simulink model "send_a429_r2019b"  (R2019b)
settings: Solver=VariableStepAuto  StartTime=0.0  StopTime=10.0  RelTol=1e-3
PreLoadFcn:
  | ds = Simulink.SimulationData.Dataset();
  | ds = ds.addElement(timeseries(uint8((1:11)' + (1:4)),       (0:10)', 'Name', 'AnA429SamplingMessage'),   'Name', 'AnA429SamplingMessage');
  | ds = ds.addElement(timeseries(uint8((250:-1:240)' + (1:4)), (0:10)', 'Name', 'AnA429QueuingMessage'),    'Name', 'AnA429QueuingMessage');
model workspace (MAT data in the model file):
  ED247Configuration(1).name = 'T11M4_A429_SIMU2SWIM_BUS_1_350_10_I'
  ED247Configuration(1).direction = 'OUT'
  ED247Configuration(1).type = 'uint8'
  ED247Configuration(1).dimensions = 1
  ED247Configuration(1).width = 4
  ED247Configuration(1).size = 4
  ED247Configuration(1).sample_time = 1
  ED247Configuration(1).validity_duration = 0
  ED247Configuration(1).signal_type = 'A429'
  ED247Configuration(1).sample_size = 4
  ED247Configuration(2).name = 'T11M4_A429_SIMU2SWIM_BUS_1_200_10_I'
  ED247Configuration(2).direction = 'OUT'
  ED247Configuration(2).type = 'uint8'
  ED247Configuration(2).dimensions = 1
  ED247Configuration(2).width = 4
  ED247Configuration(2).size = 4
  ED247Configuration(2).sample_time = 1
  ED247Configuration(2).validity_duration = 0
  ED247Configuration(2).signal_type = 'A429'
  ED247Configuration(2).sample_size = 4
  ED247Configuration(3).name = 'T11M4_A429_SIMU2SWIM_BUS_1_200_11_I'
  ED247Configuration(3).direction = 'OUT'
  ED247Configuration(3).type = 'uint8'
  ED247Configuration(3).dimensions = 1
  ED247Configuration(3).width = 4
  ED247Configuration(3).size = 4
  ED247Configuration(3).sample_time = 1
  ED247Configuration(3).validity_duration = 0
  ED247Configuration(3).signal_type = 'A429'
  ED247Configuration(3).sample_size = 4
libraries: lib_ed247 x2
settings Model: EnablePacing=on  Creator=odufour  LastModifiedBy=odufour
settings DataIOCC: ExternalInput=ds  LoadExternalInput=on

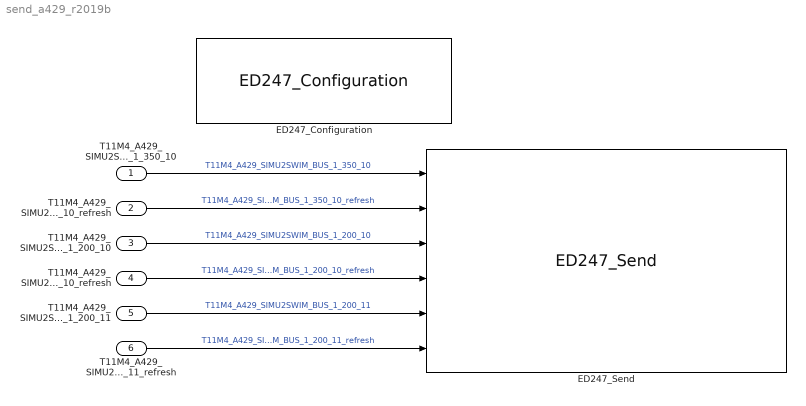
== system send_a429_r2019b ==
  T11M4_A429_SIMU2SWIM_BUS_1_350_10 : Inport  OutDataTypeStr=uint8  PortDimensions=4  SampleTime=0.1
  T11M4_A429_SIMU2SWIM_BUS_1_350_10_refresh : Inport  Port=2  OutDataTypeStr=boolean
  T11M4_A429_SIMU2SWIM_BUS_1_200_10 : Inport  Port=3  OutDataTypeStr=uint8  PortDimensions=4  SampleTime=0.1
  T11M4_A429_SIMU2SWIM_BUS_1_200_10_refresh : Inport  Port=4  OutDataTypeStr=boolean
  T11M4_A429_SIMU2SWIM_BUS_1_200_11 : Inport  Port=5  OutDataTypeStr=uint8  PortDimensions=4  SampleTime=0.1
  T11M4_A429_SIMU2SWIM_BUS_1_200_11_refresh : Inport  Port=6  OutDataTypeStr=boolean
  ED247_Configuration : lib_ed247/ED247_Configuration  configurationFilename='ecic_func_exchange_a429_uc_main_simple.xml'  enableLog=off  logFilename=''
      settings: SourceProductName=Airbus ED247
  ED247_Send : lib_ed247/ED247_Send  enable_refresh=on  show_port_labels=on
      settings: SourceProductName=Airbus ED247
  wires:
  T11M4_A429_SIMU2SWIM_BUS_1_350_10/1 -> ED247_Send/1  "T11M4_A429_SIMU2SWIM_BUS_1_350_10"
  T11M4_A429_SIMU2SWIM_BUS_1_350_10_refresh/1 -> ED247_Send/2  "T11M4_A429_SIMU2SWIM_BUS_1_350_10_refresh"
  T11M4_A429_SIMU2SWIM_BUS_1_200_10/1 -> ED247_Send/3  "T11M4_A429_SIMU2SWIM_BUS_1_200_10"
  T11M4_A429_SIMU2SWIM_BUS_1_200_10_refresh/1 -> ED247_Send/4  "T11M4_A429_SIMU2SWIM_BUS_1_200_10_refresh"
  T11M4_A429_SIMU2SWIM_BUS_1_200_11/1 -> ED247_Send/5  "T11M4_A429_SIMU2SWIM_BUS_1_200_11"
  T11M4_A429_SIMU2SWIM_BUS_1_200_11_refresh/1 -> ED247_Send/6  "T11M4_A429_SIMU2SWIM_BUS_1_200_11_refresh"
